simulink model "IntakeManifold"  (R2025b)
settings: Solver=VariableStepAuto  StartTime=0.0  StopTime=10.0  RelTol=1e-3
undefined symbols (not defined in the file or in its folder): R, Vm
settings Model: Creator=khanh  LastModifiedBy=khanh

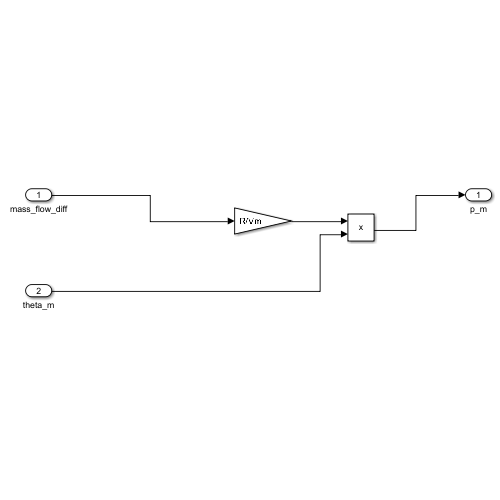
[thumbnail: Simulink's stored preview of the top-level diagram]
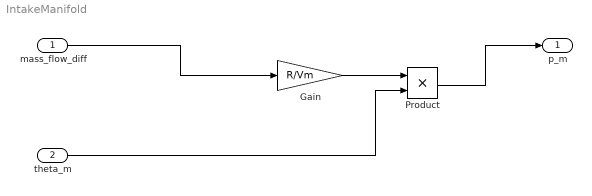
== system IntakeManifold ==
  mass_flow_diff : Inport
  theta_m : Inport  Port=2
  Gain : Gain  Gain=R/Vm
  Product : Product
  p_m : Outport
  wires:
  mass_flow_diff/1 -> Gain/1
  Gain/1 -> Product/1
  theta_m/1 -> Product/2
  Product/1 -> p_m/1
